simulink library "dkc"  (R2021b)
settings: Solver=VariableStepAuto  StartTime=0.0  StopTime=10.0  RelTol=1e-3
undefined symbols (not defined in the file or in its folder): ENUM_DKCAuthSta_DECRYPTIONFAIL, ENUM_DKCAuthSta_NORMAL, ENUM_DKCAuthSta_TIMEERROR, KDKC_DKCDecryptionErrorAllow_s, KDKC_InitialTimeErrorAllow_cnt, KDKC_TimeSNAllowDiff_cnt, ONE_INT
libraries: hcu_lib x2
settings Model: Creator=Shawn  LastModifiedBy=FVT23118
settings SolverCC: AlgebraicLoopSolver=TrustRegion
settings DebuggingCC: SFMachineParentedDataDiag=warning

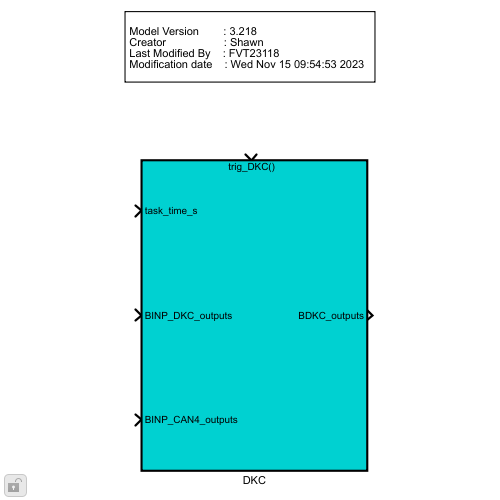
[thumbnail: Simulink's stored preview of the top-level diagram]
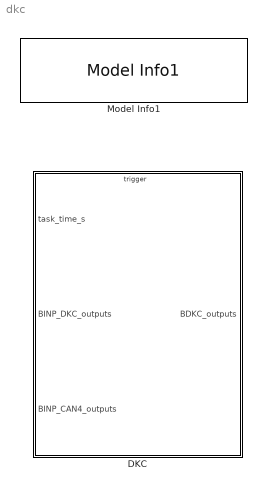
== system dkc ==
  DKC : Subsystem  TreatAsAtomicUnit=on
      settings: RTWSystemCode=Nonreusable function  RTWFcnNameOpts=Use subsystem name  RTWFileNameOpts=Use subsystem name
  Model Info1 : hcu_lib/Model Info1  BlockCM=None  Frame=on  DisplayStringWithTags=|  HorizontalTextAlignment=Left  LeftAlignmentValue=0.02  SourceBlockDiagram=hcu_lib  TagMaxNumber=20
      | Model Version        : %<ModelVersion>
      | Creator                   : %<Creator>
      | Last Modified By    : %<LastModifiedBy>
      | Modification date    : %<LastModificationDate>
      settings: SourceProductName=HCU Relative Block Library

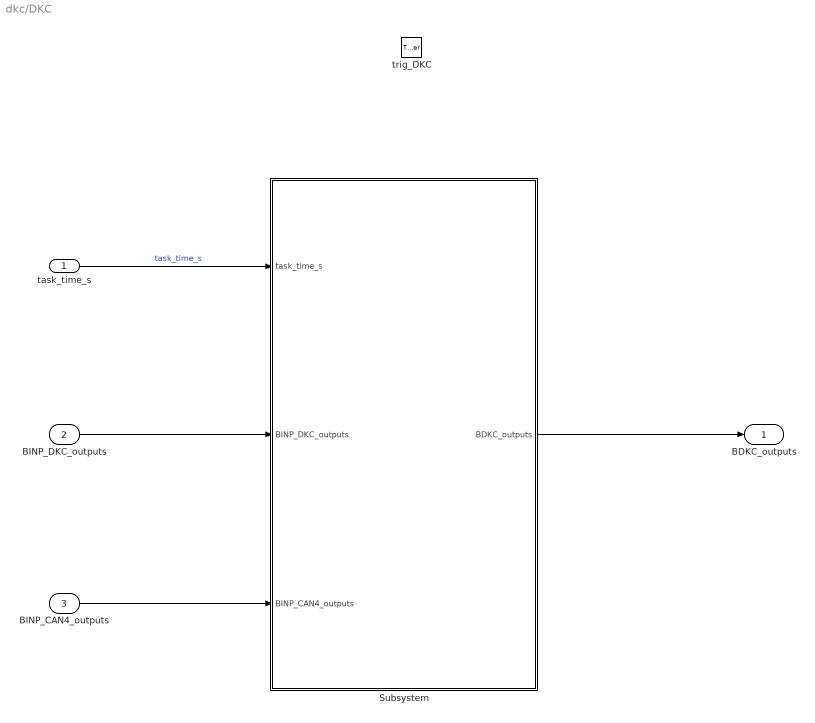
== system dkc/DKC ==
  task_time_s : Inport
  BINP_DKC_outputs : Inport  Port=2  OutDataTypeStr=Bus: BINP_DKC_outputs
  BINP_CAN4_outputs : Inport  Port=3  OutDataTypeStr=Bus: BINP_CAN4_outputs
  trig_DKC : TriggerPort  TriggerType=function-call  VariantControl=(inherit)
  Subsystem : Subsystem
  BDKC_outputs : Outport  OutDataTypeStr=Bus: BDKC_outputs
  wires:
  task_time_s/1 -> Subsystem/1(task_time_s)  "task_time_s"
  BINP_DKC_outputs/1 -> Subsystem/2(BINP_DKC_outputs)
  Subsystem/1(BDKC_outputs) -> BDKC_outputs/1
  BINP_CAN4_outputs/1 -> Subsystem/3(BINP_CAN4_outputs)

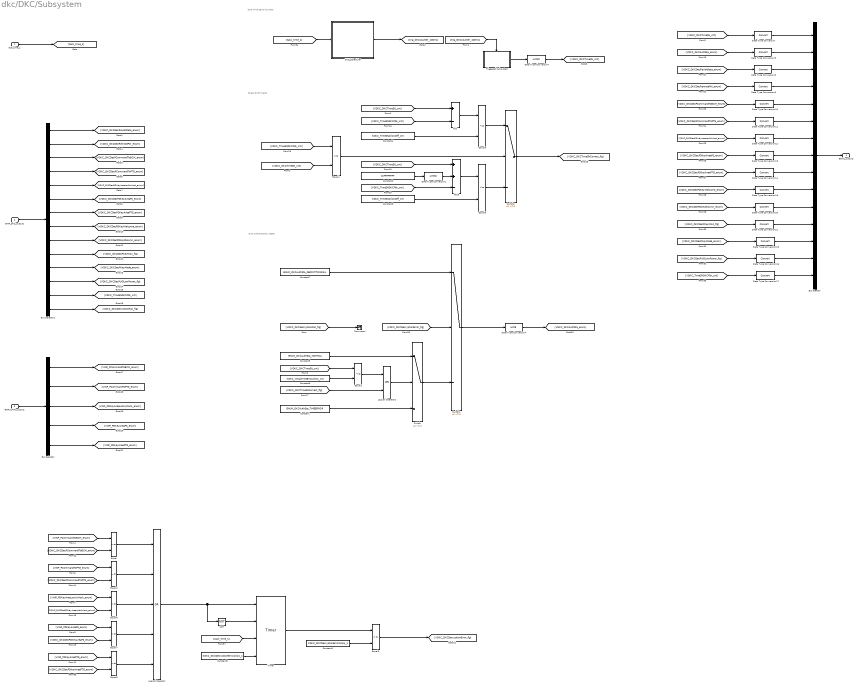
== system dkc/DKC/Subsystem ==
  note: DKC Time Serial Number
  note: Check DKCTimeSN
  note: DKC Authentication State
  task_time_s : Inport
  BINP_DKC_outputs : Inport  Port=2  OutDataTypeStr=Bus: BINP_DKC_outputs
  BINP_CAN4_outputs : Inport  Port=3  OutDataTypeStr=Bus: BINP_CAN4_outputs
  Add : Sum  Inputs=+-
  Add3 : Sum  Inputs=++-
  Bus Creator : BusCreator  Inputs=15
  Bus Selector : BusSelector  OutputSignals=VINP_PCommandToBCM_enum,VINP_PCommandToPTG_enum,VINP_PDKeyAreaLockUnlock_enum,VINP_PDKeyAreaPS_enum,VINP_PDKeyAreaPTG_enum
  Bus Selector1 : BusSelector  OutputSignals=VINP_DKCDecReVehData_enum,VINP_DKCDecRemotePW_enum,VINP_DKCDecPCommandToBCM_enum,VINP_DKCDecPCommandToPTG_enum,VINP_DKCDecPDKeyAreaLockUnlock_enum,VINP_DKCDecPDKeyAreaPS_enum,VINP_DKCDecPDKeyAreaPTG_enum,VINP_DKCDecPDKeyWelcome_enum,VINP_DKCDecPDkeyShowIVI_enum,VINP_DKCDecPKeyMiss_flg,VINP_DKCDecPKeyMode_enum,VINP_DKCDecPUIDLowPower_flg,VINP_TimeSNDKCFbk_cnt,VINP_DKCDecryptionFail_flg
  Constant : Constant  Value=ENUM_DKCAuthSta_TIMEERROR
  Constant1 : Constant  Value=KDKC_DKCDecryptionErrorAllow_s
  Constant2 : Constant  Value=0xFFFFFFFF
  Constant3 : Constant  Value=KDKC_TimeSNAllowDiff_cnt
  Constant4 : Constant  Value=KDKC_TimeSNAllowDiff_cnt
  Constant5 : Constant  Value=ENUM_DKCAuthSta_NORMAL
  Constant6 : Constant  Value=KDKC_InitialTimeErrorAllow_cnt
  Constant7 : Constant  Value=ENUM_DKCAuthSta_DECRYPTIONFAIL
  Constant8 : Constant  Value=KDKC_DKCDecryptionErrorAllow_s
  DKC_Scheduler : Stateflow chart  TreatAsAtomicUnit=on
  Data Type Conversion{,5,8..17,19..21} (15 alike) : DataTypeConversion
  Data Type Conversion1 : DataTypeConversion  OutDataTypeStr=uint32
  Data Type Conversion4 : DataTypeConversion  OutDataTypeStr=uint8
  Data Type Conversion7 : DataTypeConversion  OutDataTypeStr=uint32
  Equal{,2,6..8} (5 alike) : RelationalOperator  Operator=~=  OutDataTypeStr=boolean  RndMeth=Simplest
  Equal{1,3..5} (4 alike) : RelationalOperator  Operator=<=  OutDataTypeStr=boolean  RndMeth=Simplest
  Equal9 : RelationalOperator  OutDataTypeStr=boolean  RndMeth=Simplest
  Logical Operator : Logic  Operator=OR  Inputs=5  AllPortsSameDT=off  OutDataTypeStr=boolean
  Logical Operator1 : Logic  Operator=OR  AllPortsSameDT=off  OutDataTypeStr=boolean
  NOT : Logic  Operator=NOT  AllPortsSameDT=off  OutDataTypeStr=boolean
  Switch : Switch  Criteria=u2 ~= 0
  Switch1 : Switch  Criteria=u2 ~= 0
  Switch2 : Switch  Criteria=u2 ~= 0
  Terminator : Terminator
  Timer : hcu_lib/Basic_Blocks/Timer
  Triggered Subsystem : Subsystem  TreatAsAtomicUnit=on
  BDKC_outputs : Outport
  wires:
  task_time_s/1 -> [task_time_s]
  DKC_Scheduler/1(trig_DKCcounter_100ms()) -> [trig_DKCcounter_100ms]
  [trig_DKCcounter_100ms] -> Triggered Subsystem/Trigger
  BINP_DKC_outputs/1 -> Bus Selector1/1
  [VDKC_TimeSNDKCFbk_cnt] -> Add/2
  Add/1 -> Equal3/1
  Constant4/1 -> Equal3/2
  [VDKC_TimeSNDKCFbk_cnt] -> Equal4/1
  Equal4/1 -> Switch2/2
  Equal3/1 -> Switch2/1
  Equal5/1 -> Switch2/3
  [task_time_s] -> DKC_Scheduler/1(task_time_s)
  Switch2/1 -> [VDKC_DKCTimeSNCorrect_flg]  "VDKC_DKCTimeSNCorrect_flg"
  Triggered Subsystem/1(DKCTimeSN) -> Data Type Conversion7/1
  Data Type Conversion7/1 -> [VDKC_DKCTimeSN_cnt]
  [VDKC_DKCTimeSN_cnt] -> Add/1
  Bus Selector1/1 -> [VDKC_DKCDecReVehData_enum]  "<VINP_DKCDecReVehData_enum>"
  Bus Selector1/2 -> [VDKC_DKCDecRemotePW_enum]  "<VINP_DKCDecRemotePW_enum>"
  Bus Selector1/3 -> [VDKC_DKCDecPCommandToBCM_enum]  "<VINP_DKCDecPCommandToBCM_enum>"
  Bus Selector1/4 -> [VDKC_DKCDecPCommandToPTG_enum]  "<VINP_DKCDecPCommandToPTG_enum>"
  Bus Selector1/5 -> [VDKC_DKCDecPDKeyAreaLockUnlock_enum]  "<VINP_DKCDecPDKeyAreaLockUnlock_enum>"
  Bus Selector1/6 -> [VDKC_DKCDecPDKeyAreaPS_enum]  "<VINP_DKCDecPDKeyAreaPS_enum>"
  Bus Selector1/7 -> [VDKC_DKCDecPDKeyAreaPTG_enum]  "<VINP_DKCDecPDKeyAreaPTG_enum>"
  Bus Selector1/8 -> [VDKC_DKCDecPDKeyWelcome_enum]  "<VINP_DKCDecPDKeyWelcome_enum>"
  Bus Selector1/9 -> [VDKC_DKCDecPDkeyShowIVI_enum]  "<VINP_DKCDecPDkeyShowIVI_enum>"
  Bus Selector1/10 -> [VDKC_DKCDecPKeyMiss_flg]  "<VINP_DKCDecPKeyMiss_flg>"
  Bus Selector1/11 -> [VDKC_DKCDecPKeyMode_enum]  "<VINP_DKCDecPKeyMode_enum>"
  Bus Selector1/12 -> [VDKC_DKCDecPUIDLowPower_flg]  "<VINP_DKCDecPUIDLowPower_flg>"
  Bus Selector1/13 -> [VDKC_TimeSNDKCFbk_cnt]  "<VINP_TimeSNDKCFbk_cnt>"
  Bus Creator/1 -> BDKC_outputs/1  "BDKC_outputs"
  Data Type Conversion/1 -> Bus Creator/1  "VDKC_DKCTimeSN_cnt"
  [VDKC_DKCTimeSN_cnt] -> Data Type Conversion/1
  Data Type Conversion15/1 -> Bus Creator/13  "VDKC_DKCDecPKeyMode_enum"
  Data Type Conversion13/1 -> Bus Creator/8  "VDKC_DKCDecPDKeyAreaPS_enum"
  [VDKC_DKCDecPDKeyAreaLockUnlock_enum] -> Data Type Conversion12/1
  Data Type Conversion20/1 -> Bus Creator/11  "VDKC_DKCDecPDkeyShowIVI_enum"
  Data Type Conversion11/1 -> Bus Creator/6  "VDKC_DKCDecPCommandToPTG_enum"
  [VDKC_TimeSNDKCFbk_cnt] -> Data Type Conversion17/1
  Data Type Conversion21/1 -> Bus Creator/12  "VDKC_DKCDecPKeyMiss_flg"
  [VDKC_DKCDecPDKeyAreaPS_enum] -> Data Type Conversion13/1
  Data Type Conversion17/1 -> Bus Creator/15  "VDKC_TimeSNDKCFbk_cnt"
  [VDKC_DKCDecPKeyMiss_flg] -> Data Type Conversion21/1
  [VDKC_DKCDecPDkeyShowIVI_enum] -> Data Type Conversion20/1
  [VDKC_DKCDecPCommandToPTG_enum] -> Data Type Conversion11/1
  [VDKC_DKCDecPDKeyAreaPTG_enum] -> Data Type Conversion14/1
  [VDKC_DKCDecPKeyMode_enum] -> Data Type Conversion15/1
  [VDKC_DKCDecPUIDLowPower_flg] -> Data Type Conversion16/1
  [VDKC_DKCDecPDKeyWelcome_enum] -> Data Type Conversion19/1
  [VDKC_DKCDecRemotePW_enum] -> Data Type Conversion9/1
  Data Type Conversion19/1 -> Bus Creator/10  "VDKC_DKCDecPDKeyWelcome_enum"
  [VDKC_DKCDecPCommandToBCM_enum] -> Data Type Conversion10/1
  Data Type Conversion8/1 -> Bus Creator/3  "VDKC_DKCDecReVehData_enum"
  Data Type Conversion5/1 -> Bus Creator/2  "VDKC_DKCAuthSta_enum"
  Data Type Conversion14/1 -> Bus Creator/9  "VDKC_DKCDecPDKeyAreaPTG_enum"
  Data Type Conversion12/1 -> Bus Creator/7  "VDKC_DKCDecPDKeyAreaLockUnlock_enum"
  [VDKC_DKCDecReVehData_enum] -> Data Type Conversion8/1
  Data Type Conversion9/1 -> Bus Creator/4  "VDKC_DKCDecRemotePW_enum"
  Data Type Conversion10/1 -> Bus Creator/5  "VDKC_DKCDecPCommandToBCM_enum"
  Data Type Conversion16/1 -> Bus Creator/14  "VDKC_DKCDecPUIDLowPower_flg"
  [VDKC_DKCAuthSta_enum] -> Data Type Conversion5/1
  [VDKC_DKCTimeSN_cnt] -> Equal4/2
  [VDKC_DKCTimeSN_cnt] -> Add3/1
  Constant2/1 -> Data Type Conversion1/1
  Data Type Conversion1/1 -> Add3/2
  Add3/1 -> Equal5/1
  [VDKC_TimeSNDKCFbk_cnt] -> Add3/3
  Constant3/1 -> Equal5/2
  Constant/1 -> Switch/3
  Constant5/1 -> Switch/1
  Logical Operator1/1 -> Switch/2
  Equal1/1 -> Logical Operator1/1
  Switch/1 -> Switch1/3
  Data Type Conversion4/1 -> [VDKC_DKCAuthSta_enum]
  Constant7/1 -> Switch1/1
  [VDKC_DKCTimeSN_cnt] -> Equal1/1
  [VDKC_DKCTimeSNCorrect_flg] -> Logical Operator1/2
  Constant6/1 -> Equal1/2
  Switch1/1 -> Data Type Conversion4/1
  Bus Selector1/14 -> [VDKC_DKCDecryptionFail_flg]  "<VINP_DKCDecryptionFail_flg>"
  BINP_CAN4_outputs/1 -> Bus Selector/1
  Bus Selector/1 -> [VINP_PCommandToBCM_enum]  "<VINP_PCommandToBCM_enum>"
  Bus Selector/2 -> [VINP_PCommandToPTG_enum]  "<VINP_PCommandToPTG_enum>"
  Bus Selector/3 -> [VINP_PDKeyAreaLockUnlock_enum]  "<VINP_PDKeyAreaLockUnlock_enum>"
  Bus Selector/4 -> [VINP_PDKeyAreaPS_enum]  "<VINP_PDKeyAreaPS_enum>"
  Bus Selector/5 -> [VINP_PDKeyAreaPTG_enum]  "<VINP_PDKeyAreaPTG_enum>"
  [VINP_PCommandToBCM_enum] -> Equal/1
  [VDKC_DKCDecPCommandToBCM_enum] -> Equal/2
  [VINP_PCommandToPTG_enum] -> Equal2/1
  [VDKC_DKCDecPCommandToPTG_enum] -> Equal2/2
  [VINP_PDKeyAreaPS_enum] -> Equal7/1
  [VINP_PDKeyAreaPTG_enum] -> Equal8/1
  [VDKC_DKCDecPDKeyAreaPS_enum] -> Equal7/2
  [VDKC_DKCDecPDKeyAreaLockUnlock_enum] -> Equal6/2
  [VINP_PDKeyAreaLockUnlock_enum] -> Equal6/1
  [VDKC_DKCDecPDKeyAreaPTG_enum] -> Equal8/2
  Equal2/1 -> Logical Operator/2
  Equal6/1 -> Logical Operator/3
  Equal/1 -> Logical Operator/1
  Equal7/1 -> Logical Operator/4
  Equal8/1 -> Logical Operator/5
  [VDKC_DKCDecryptionFail_flg] -> Terminator/1
  [VDKC_DKCDecryptionError_flg] -> Switch1/2
  Logical Operator/1 -> Timer/1, NOT/1
  Timer/1 -> Equal9/1
  Constant1/1 -> Equal9/2
  Equal9/1 -> [VDKC_DKCDecryptionError_flg]  "VDKC_DKCDecryptionError_flg"
  NOT/1 -> Timer/2
  [task_time_s] -> Timer/3
  Constant8/1 -> Timer/4

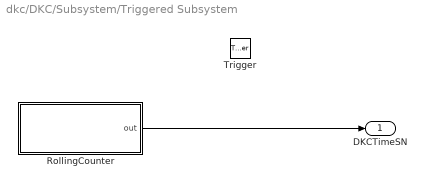
== system dkc/DKC/Subsystem/Triggered Subsystem ==
  Trigger : TriggerPort  TriggerType=function-call  VariantControl=(inherit)
  RollingCounter : Subsystem  mask{CounterMAX=4294967295}
      mask help: MeasumentTrigerEvent
      mask Display: fprintf('RollingCounter');
  DKCTimeSN : Outport
  wires:
  RollingCounter/1(out) -> DKCTimeSN/1

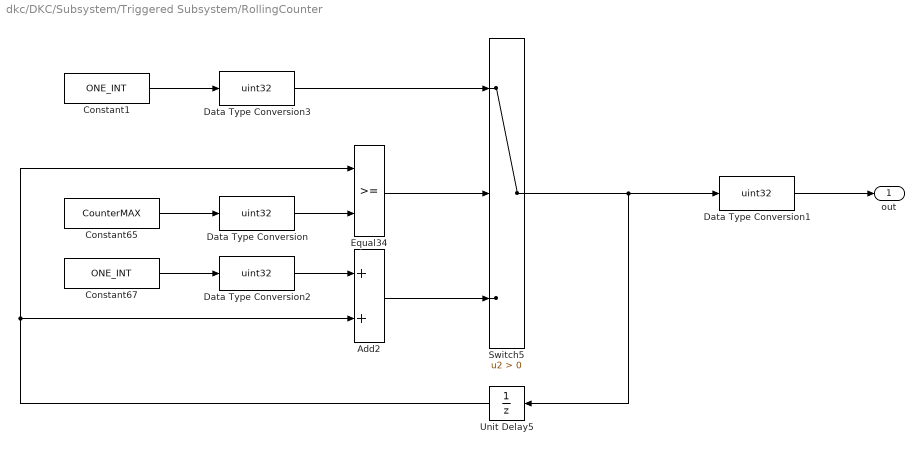
== system dkc/DKC/Subsystem/Triggered Subsystem/RollingCounter ==
  Add2 : Sum
  Constant1 : Constant  Value=ONE_INT
  Constant65 : Constant  Value=CounterMAX
  Constant67 : Constant  Value=ONE_INT
  Data Type Conversion{,1..3} (4 alike) : DataTypeConversion  OutDataTypeStr=uint32
  Equal34 : RelationalOperator  OutDataTypeStr=boolean  RndMeth=Simplest
  Switch5 : Switch  Criteria=u2 > Threshold
  Unit Delay5 : UnitDelay  SampleTime=-1  HasFrameUpgradeWarning=on
  out : Outport
  wires:
  Data Type Conversion1/1 -> out/1
  Constant65/1 -> Data Type Conversion/1
  Data Type Conversion/1 -> Equal34/2
  Unit Delay5/1 -> Equal34/1, Add2/2
  Constant67/1 -> Data Type Conversion2/1
  Add2/1 -> Switch5/3
  Constant1/1 -> Data Type Conversion3/1
  Equal34/1 -> Switch5/2
  Switch5/1 -> Unit Delay5/1, Data Type Conversion1/1
  Data Type Conversion2/1 -> Add2/1
  Data Type Conversion3/1 -> Switch5/1

== stateflow chart dkc/DKC/Subsystem/DKC_Scheduler ==
  state trigger_100ms
    (default) -> (junction 1) : {
        | counter = 0;
        | }
    trigger_100ms -> (junction 1) : {
        | counter++;
        | }
    (junction 1) -> (junction 8) [order 1] : [counter%%uint8((0.1/task_time_s)) == 0]  /* 100ms trigger */
    (junction 1) -> (junction 5) [order 2]
    (junction 8) -> (junction 9) : {
        | trig_DKCcounter_100ms;
        | counter = 0;
        | }
    (junction 9) -> (junction 5)
  data: counter local uint32 size=1; task_time_s input
  events: trig_DKCcounter_100ms output FUNCTION_CALL_EVENT
